simulink model "SecRwRtStCaller"  (R2018b)
settings: Solver=FixedStepDiscrete  StartTime=0.0  StopTime=10.0  RelTol=1e-3
undefined symbols (not defined in the file or in its folder): SecRwRtStArmScrnCtrl_1_Cal, SecRwRtStArmScrnHolderChk_1_Cal, SecRwRtStArmScrnIsPosChk_1_Cal, SecRwRtStArmScrnTrgtPosSelc_1_Cal, SecRwRtStBkReclnCtrl_1_Cal, SecRwRtStBkReclnHolderChk_1_Cal, SecRwRtStBkReclnIsPosChk_1_Cal, SecRwRtStBkReclnTrgtPosSelc_1_Cal, SecRwRtStChldLckChk_Cal, SecRwRtStFtrstCtrl_1_Cal, SecRwRtStFtrstHolderChk_1_Cal, SecRwRtStFtrstIsPosChk_1_Cal, SecRwRtStFtrstTrgtPosSelc_1_Cal, SecRwRtStFwdBkwdCtrl_1_Cal, SecRwRtStFwdBkwdHolderChk_1_Cal, SecRwRtStFwdBkwdIsPosChk_1_Cal, SecRwRtStFwdBkwdSpdCtrl_1_Cal, SecRwRtStFwdBkwdTrgtPosSelc_1_Cal, SecRwRtStHdrstFwdBkwdCtrl_1_Cal, SecRwRtStHdrstFwdBkwdHolderChk_1_Cal, SecRwRtStHdrstFwdBkwdIsPosChk_1_Cal, SecRwRtStHdrstFwdBkwdTrgtPosSelc_1_Cal, SecRwRtStHdrstUpwdDnwdCtrl_1_Cal, SecRwRtStHdrstUpwdDnwdHolderChk_1_Cal, SecRwRtStHdrstUpwdDnwdIsPosChk_1_Cal, SecRwRtStHdrstUpwdDnwdTrgtPosSelc_1_Cal, SecRwRtStHeightChk_Cal, SecRwRtStLgrstInwdOtwdCtrl_1_Cal, SecRwRtStLgrstInwdOtwdHolderChk_1_Cal, SecRwRtStLgrstInwdOtwdIsPosChk_1_Cal, SecRwRtStLgrstInwdOtwdTrgtPosSelc_1_Cal, SecRwRtStLgrstUpwdDnwdCtrl_1_Cal, SecRwRtStLgrstUpwdDnwdHolderChk_1_Cal, SecRwRtStLgrstUpwdDnwdIsPosChk_1_Cal, SecRwRtStLgrstUpwdDnwdTrgtPosSelc_1_Cal, SecRwRtStLtwdRtwdCtrl_1_Cal, SecRwRtStLtwdRtwdHolderChk_1_Cal, SecRwRtStLtwdRtwdIsPosChk_1_Cal, SecRwRtStLtwdRtwdTrgtPosSelc_1_Cal, SecRwRtStOccupyChk_Cal, SecRwRtStRclCmdSrvCal_1_Cal, SecRwRtStZeroCtrl_1_Cal, SecRwRtStZeroHolderChk_1_Cal, SecRwRtStZeroIsPosChk_1_Cal, SecRwRtStZeroTrgtPosSelc_1_Cal
settings Model: Creator=sn2xws  LastModifiedBy=sn2xws
settings Model: ModifiedHistory=|
  | 2024.5.6
  | 557 新增零重力电机
settings DataIOCC: SaveFormat=StructureWithTime
settings OptimizationCC: DefaultParameterBehavior=Inlined  EnhancedBackFolding=on  PassReuseOutputArgsAs=Individual arguments  ZeroExternalMemoryAtStartup=off  ZeroInternalMemoryAtStartup=off  OptimizeBlockOrder=speed  DifferentSizesBufferReuse=on  OptimizationCustomize=off
settings DebuggingCC: ParameterTunabilityLossMsg=error
settings SFSimCC: MATLABDynamicMemAlloc=off
settings RTWCC: SystemTargetFile=autosar.tlc  GenCodeOnly=on  TemplateMakefile=ert_default_tmf  Description=AUTOSAR  GenerateReport=on  IncludeHyperlinkInReport=on  LaunchReport=on  GenerateTraceInfo=on  GenerateTraceReport=on  GenerateTraceReportSl=on  GenerateTraceReportSf=on  GenerateTraceReportEml=on
settings CodeAppCC: ForceParamTrailComments=on  IgnoreCustomStorageClasses=off  OperatorAnnotations=on  SimulinkDataObjDesc=on  SFDataObjDesc=on  InsertBlockDesc=on
settings STFCustomTargetCC: TargetLangStandard=C99 (ISO)  MultiwordLength=256  ParMdlRefBuildCompliant=on  CompOptLevelCompliant=on  IncludeMdlTerminateFcn=off  CombineOutputUpdateFcns=on  SuppressErrorStatus=on  ERTCustomFileBanners=on  SupportNonFinite=off  SupportComplex=off  SupportContinuousTime=off  SupportNonInlinedSFcns=off  RemoveResetFunc=on  MATLABClassNameForMDSCustomization=Simulink.SoftwareTarget.ERTCustomization  AutosarCompliant=on  UseToolchainInfoCompliant=on  LookupTableObjectStructAxisOrder=2,1,3,4,...  LUTObjectStructOrderEvenSpacing=Size,Table,Breakpoints  SystemTargetFile=autosar.tlc
settings ERTTargetCC: TargetLangStandard=C99 (ISO)  ConcurrentExecutionCompliant=off  IncludeMdlTerminateFcn=off  SuppressErrorStatus=on  SupportNonFinite=off  SupportComplex=off  ModelStepFunctionPrototypeControlCompliant=off  CPPClassGenCompliant=off  AutosarCompliant=on  LookupTableObjectStructAxisOrder=2,1,3,4,...  LUTObjectStructOrderEvenSpacing=Size,Table,Breakpoints  InlinedParameterPlacement=NonHierarchical  ERTCustomFileTemplate=example_file_process.tlc  ERTFilePackagingFormat=Compact

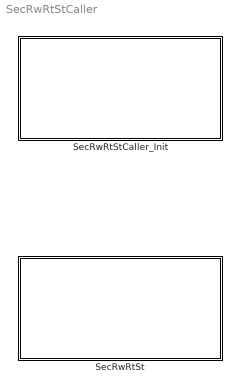
== system SecRwRtStCaller ==
  SecRwRtSt : Subsystem
  SecRwRtStCaller_Init : Subsystem

== system SecRwRtStCaller/SecRwRtSt ==
  SecRwRtSt_Cal_sys : Subsystem

== system SecRwRtStCaller/SecRwRtStCaller_Init ==
  Event Listener : EventListener  EventName=reset

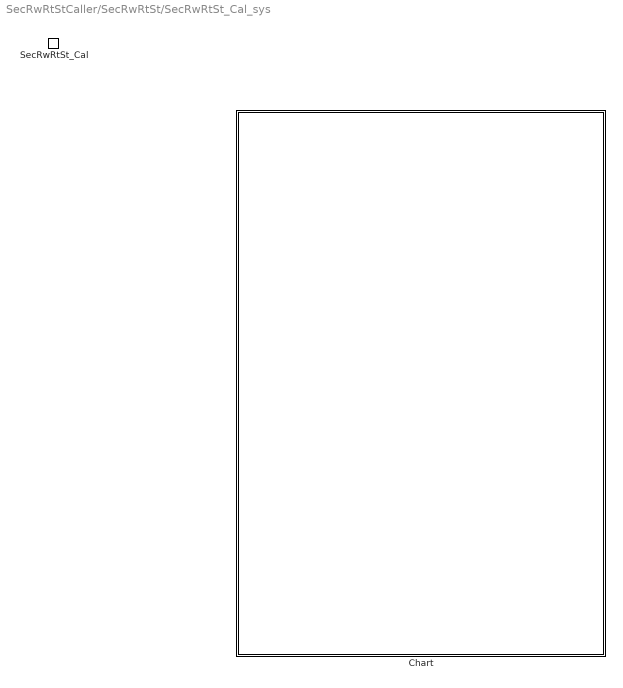
== system SecRwRtStCaller/SecRwRtSt/SecRwRtSt_Cal_sys ==
  SecRwRtSt_Cal : TriggerPort  TriggerType=function-call  IsSimulinkFunction=on  FunctionName=SecRwRtSt_Cal  VariantControl=(inherit)
  Chart : Stateflow chart  TreatAsAtomicUnit=on

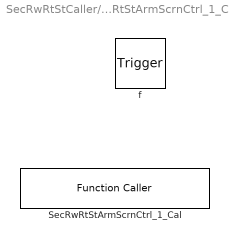
== system SecRwRtStCaller/SecRwRtSt/SecRwRtSt_Cal_sys/Chart/SecRwRtStArmScrnCtrl_1_Cal ==
  f : TriggerPort  TriggerType=function-call  VariantControl=(inherit)
      settings: CopyFcn=Stateflow.SLINSF.SimulinkMan.removeBlockPreDeleteFcn  PreDeleteFcn=Stateflow.SLINSF.SimulinkMan.unsafePredeleteFcn
  SecRwRtStArmScrnCtrl_1_Cal : FunctionCaller  FunctionPrototype=SecRwRtStArmScrnCtrl_1_Cal()

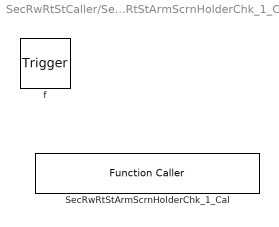
== system SecRwRtStCaller/SecRwRtSt/SecRwRtSt_Cal_sys/Chart/SecRwRtStArmScrnHolderChk_1_Cal ==
  f : TriggerPort  TriggerType=function-call  VariantControl=(inherit)
      settings: CopyFcn=Stateflow.SLINSF.SimulinkMan.removeBlockPreDeleteFcn  PreDeleteFcn=Stateflow.SLINSF.SimulinkMan.unsafePredeleteFcn
  SecRwRtStArmScrnHolderChk_1_Cal : FunctionCaller  FunctionPrototype=SecRwRtStArmScrnHolderChk_1_Cal()

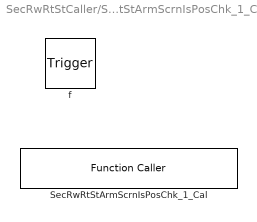
== system SecRwRtStCaller/SecRwRtSt/SecRwRtSt_Cal_sys/Chart/SecRwRtStArmScrnIsPosChk_1_Cal ==
  f : TriggerPort  TriggerType=function-call  VariantControl=(inherit)
      settings: CopyFcn=Stateflow.SLINSF.SimulinkMan.removeBlockPreDeleteFcn  PreDeleteFcn=Stateflow.SLINSF.SimulinkMan.unsafePredeleteFcn
  SecRwRtStArmScrnIsPosChk_1_Cal : FunctionCaller  FunctionPrototype=SecRwRtStArmScrnIsPosChk_1_Cal()

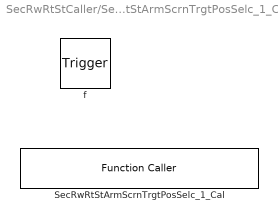
== system SecRwRtStCaller/SecRwRtSt/SecRwRtSt_Cal_sys/Chart/SecRwRtStArmScrnTrgtPosSelc_1_Cal ==
  f : TriggerPort  TriggerType=function-call  VariantControl=(inherit)
      settings: CopyFcn=Stateflow.SLINSF.SimulinkMan.removeBlockPreDeleteFcn  PreDeleteFcn=Stateflow.SLINSF.SimulinkMan.unsafePredeleteFcn
  SecRwRtStArmScrnTrgtPosSelc_1_Cal : FunctionCaller  FunctionPrototype=SecRwRtStArmScrnTrgtPosSelc_1_Cal()

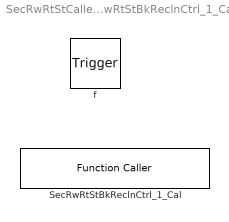
== system SecRwRtStCaller/SecRwRtSt/SecRwRtSt_Cal_sys/Chart/SecRwRtStBkReclnCtrl_1_Cal ==
  f : TriggerPort  TriggerType=function-call  VariantControl=(inherit)
      settings: CopyFcn=Stateflow.SLINSF.SimulinkMan.removeBlockPreDeleteFcn  PreDeleteFcn=Stateflow.SLINSF.SimulinkMan.unsafePredeleteFcn
  SecRwRtStBkReclnCtrl_1_Cal : FunctionCaller  FunctionPrototype=SecRwRtStBkReclnCtrl_1_Cal()

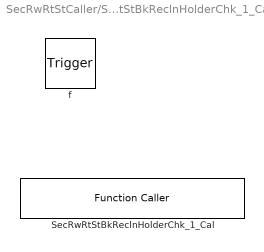
== system SecRwRtStCaller/SecRwRtSt/SecRwRtSt_Cal_sys/Chart/SecRwRtStBkReclnHolderChk_1_Cal ==
  f : TriggerPort  TriggerType=function-call  VariantControl=(inherit)
      settings: CopyFcn=Stateflow.SLINSF.SimulinkMan.removeBlockPreDeleteFcn  PreDeleteFcn=Stateflow.SLINSF.SimulinkMan.unsafePredeleteFcn
  SecRwRtStBkReclnHolderChk_1_Cal : FunctionCaller  FunctionPrototype=SecRwRtStBkReclnHolderChk_1_Cal()

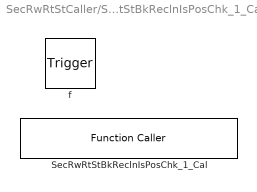
== system SecRwRtStCaller/SecRwRtSt/SecRwRtSt_Cal_sys/Chart/SecRwRtStBkReclnIsPosChk_1_Cal ==
  f : TriggerPort  TriggerType=function-call  VariantControl=(inherit)
      settings: CopyFcn=Stateflow.SLINSF.SimulinkMan.removeBlockPreDeleteFcn  PreDeleteFcn=Stateflow.SLINSF.SimulinkMan.unsafePredeleteFcn
  SecRwRtStBkReclnIsPosChk_1_Cal : FunctionCaller  FunctionPrototype=SecRwRtStBkReclnIsPosChk_1_Cal()

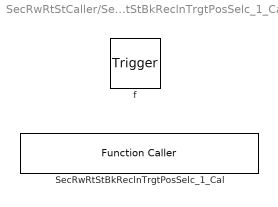
== system SecRwRtStCaller/SecRwRtSt/SecRwRtSt_Cal_sys/Chart/SecRwRtStBkReclnTrgtPosSelc_1_Cal ==
  f : TriggerPort  TriggerType=function-call  VariantControl=(inherit)
      settings: CopyFcn=Stateflow.SLINSF.SimulinkMan.removeBlockPreDeleteFcn  PreDeleteFcn=Stateflow.SLINSF.SimulinkMan.unsafePredeleteFcn
  SecRwRtStBkReclnTrgtPosSelc_1_Cal : FunctionCaller  FunctionPrototype=SecRwRtStBkReclnTrgtPosSelc_1_Cal()

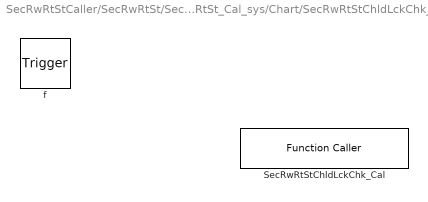
== system SecRwRtStCaller/SecRwRtSt/SecRwRtSt_Cal_sys/Chart/SecRwRtStChldLckChk_Cal ==
  f : TriggerPort  TriggerType=function-call  VariantControl=(inherit)
      settings: CopyFcn=Stateflow.SLINSF.SimulinkMan.removeBlockPreDeleteFcn  PreDeleteFcn=Stateflow.SLINSF.SimulinkMan.unsafePredeleteFcn
  SecRwRtStChldLckChk_Cal : FunctionCaller  FunctionPrototype=SecRwRtStChldLckChk_Cal()

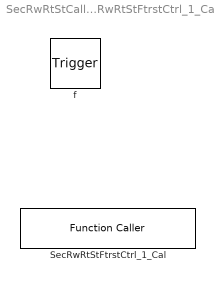
== system SecRwRtStCaller/SecRwRtSt/SecRwRtSt_Cal_sys/Chart/SecRwRtStFtrstCtrl_1_Cal ==
  f : TriggerPort  TriggerType=function-call  VariantControl=(inherit)
      settings: CopyFcn=Stateflow.SLINSF.SimulinkMan.removeBlockPreDeleteFcn  PreDeleteFcn=Stateflow.SLINSF.SimulinkMan.unsafePredeleteFcn
  SecRwRtStFtrstCtrl_1_Cal : FunctionCaller  FunctionPrototype=SecRwRtStFtrstCtrl_1_Cal()

== system SecRwRtStCaller/SecRwRtSt/SecRwRtSt_Cal_sys/Chart/SecRwRtStFtrstHolderChk_1_Cal ==
  f : TriggerPort  TriggerType=function-call  VariantControl=(inherit)
      settings: CopyFcn=Stateflow.SLINSF.SimulinkMan.removeBlockPreDeleteFcn  PreDeleteFcn=Stateflow.SLINSF.SimulinkMan.unsafePredeleteFcn
  SecRwRtStFtrstHolderChk_1_Cal : FunctionCaller  FunctionPrototype=SecRwRtStFtrstHolderChk_1_Cal()

== system SecRwRtStCaller/SecRwRtSt/SecRwRtSt_Cal_sys/Chart/SecRwRtStFtrstIsPosChk_1_Cal ==
  f : TriggerPort  TriggerType=function-call  VariantControl=(inherit)
      settings: CopyFcn=Stateflow.SLINSF.SimulinkMan.removeBlockPreDeleteFcn  PreDeleteFcn=Stateflow.SLINSF.SimulinkMan.unsafePredeleteFcn
  SecRwRtStFtrstIsPosChk_1_Cal : FunctionCaller  FunctionPrototype=SecRwRtStFtrstIsPosChk_1_Cal()

== system SecRwRtStCaller/SecRwRtSt/SecRwRtSt_Cal_sys/Chart/SecRwRtStFtrstTrgtPosSelc_1_Cal ==
  f : TriggerPort  TriggerType=function-call  VariantControl=(inherit)
      settings: CopyFcn=Stateflow.SLINSF.SimulinkMan.removeBlockPreDeleteFcn  PreDeleteFcn=Stateflow.SLINSF.SimulinkMan.unsafePredeleteFcn
  SecRwRtStFtrstTrgtPosSelc_1_Cal : FunctionCaller  FunctionPrototype=SecRwRtStFtrstTrgtPosSelc_1_Cal()

== system SecRwRtStCaller/SecRwRtSt/SecRwRtSt_Cal_sys/Chart/SecRwRtStFwdBkwdCtrl_1_Cal ==
  f : TriggerPort  TriggerType=function-call  VariantControl=(inherit)
      settings: CopyFcn=Stateflow.SLINSF.SimulinkMan.removeBlockPreDeleteFcn  PreDeleteFcn=Stateflow.SLINSF.SimulinkMan.unsafePredeleteFcn
  SecRwRtStFwdBkwdCtrl_1_Cal : FunctionCaller  FunctionPrototype=SecRwRtStFwdBkwdCtrl_1_Cal()

== system SecRwRtStCaller/SecRwRtSt/SecRwRtSt_Cal_sys/Chart/SecRwRtStFwdBkwdHolderChk_1_Cal ==
  f : TriggerPort  TriggerType=function-call  VariantControl=(inherit)
      settings: CopyFcn=Stateflow.SLINSF.SimulinkMan.removeBlockPreDeleteFcn  PreDeleteFcn=Stateflow.SLINSF.SimulinkMan.unsafePredeleteFcn
  SecRwRtStFwdBkwdHolderChk_1_Cal : FunctionCaller  FunctionPrototype=SecRwRtStFwdBkwdHolderChk_1_Cal()

== system SecRwRtStCaller/SecRwRtSt/SecRwRtSt_Cal_sys/Chart/SecRwRtStFwdBkwdIsPosChk_1_Cal ==
  f : TriggerPort  TriggerType=function-call  VariantControl=(inherit)
      settings: CopyFcn=Stateflow.SLINSF.SimulinkMan.removeBlockPreDeleteFcn  PreDeleteFcn=Stateflow.SLINSF.SimulinkMan.unsafePredeleteFcn
  SecRwRtStFwdBkwdIsPosChk_1_Cal : FunctionCaller  FunctionPrototype=SecRwRtStFwdBkwdIsPosChk_1_Cal()

== system SecRwRtStCaller/SecRwRtSt/SecRwRtSt_Cal_sys/Chart/SecRwRtStFwdBkwdSpdCtrl_1_Cal ==
  f : TriggerPort  TriggerType=function-call  VariantControl=(inherit)
      settings: CopyFcn=Stateflow.SLINSF.SimulinkMan.removeBlockPreDeleteFcn  PreDeleteFcn=Stateflow.SLINSF.SimulinkMan.unsafePredeleteFcn
  SecRwRtStFwdBkwdSpdCtrl_1_Cal : FunctionCaller  FunctionPrototype=SecRwRtStFwdBkwdSpdCtrl_1_Cal()

== system SecRwRtStCaller/SecRwRtSt/SecRwRtSt_Cal_sys/Chart/SecRwRtStFwdBkwdTrgtPosSelc_1_Cal ==
  f : TriggerPort  TriggerType=function-call  VariantControl=(inherit)
      settings: CopyFcn=Stateflow.SLINSF.SimulinkMan.removeBlockPreDeleteFcn  PreDeleteFcn=Stateflow.SLINSF.SimulinkMan.unsafePredeleteFcn
  SecRwRtStFwdBkwdTrgtPosSelc_1_Cal : FunctionCaller  FunctionPrototype=SecRwRtStFwdBkwdTrgtPosSelc_1_Cal()

== system SecRwRtStCaller/SecRwRtSt/SecRwRtSt_Cal_sys/Chart/SecRwRtStHdrstFwdBkwdCtrl_1_Cal ==
  f : TriggerPort  TriggerType=function-call  VariantControl=(inherit)
      settings: CopyFcn=Stateflow.SLINSF.SimulinkMan.removeBlockPreDeleteFcn  PreDeleteFcn=Stateflow.SLINSF.SimulinkMan.unsafePredeleteFcn
  SecRwRtStHdrstFwdBkwdCtrl_1_Cal : FunctionCaller  FunctionPrototype=SecRwRtStHdrstFwdBkwdCtrl_1_Cal()

== system SecRwRtStCaller/SecRwRtSt/SecRwRtSt_Cal_sys/Chart/SecRwRtStHdrstFwdBkwdHolderChk_1_Cal ==
  f : TriggerPort  TriggerType=function-call  VariantControl=(inherit)
      settings: CopyFcn=Stateflow.SLINSF.SimulinkMan.removeBlockPreDeleteFcn  PreDeleteFcn=Stateflow.SLINSF.SimulinkMan.unsafePredeleteFcn
  SecRwRtStHdrstFwdBkwdHolderChk_1_Cal : FunctionCaller  FunctionPrototype=SecRwRtStHdrstFwdBkwdHolderChk_1_Cal()

== system SecRwRtStCaller/SecRwRtSt/SecRwRtSt_Cal_sys/Chart/SecRwRtStHdrstFwdBkwdIsPosChk_1_Cal ==
  f : TriggerPort  TriggerType=function-call  VariantControl=(inherit)
      settings: CopyFcn=Stateflow.SLINSF.SimulinkMan.removeBlockPreDeleteFcn  PreDeleteFcn=Stateflow.SLINSF.SimulinkMan.unsafePredeleteFcn
  SecRwRtStHdrstFwdBkwdIsPosChk_1_Cal : FunctionCaller  FunctionPrototype=SecRwRtStHdrstFwdBkwdIsPosChk_1_Cal()

== system SecRwRtStCaller/SecRwRtSt/SecRwRtSt_Cal_sys/Chart/SecRwRtStHdrstFwdBkwdTrgtPosSelc_1_Cal ==
  f : TriggerPort  TriggerType=function-call  VariantControl=(inherit)
      settings: CopyFcn=Stateflow.SLINSF.SimulinkMan.removeBlockPreDeleteFcn  PreDeleteFcn=Stateflow.SLINSF.SimulinkMan.unsafePredeleteFcn
  SecRwRtStHdrstFwdBkwdTrgtPosSelc_1_Cal : FunctionCaller  FunctionPrototype=SecRwRtStHdrstFwdBkwdTrgtPosSelc_1_Cal()

== system SecRwRtStCaller/SecRwRtSt/SecRwRtSt_Cal_sys/Chart/SecRwRtStHdrstUpwdDnwdCtrl_1_Cal ==
  f : TriggerPort  TriggerType=function-call  VariantControl=(inherit)
      settings: CopyFcn=Stateflow.SLINSF.SimulinkMan.removeBlockPreDeleteFcn  PreDeleteFcn=Stateflow.SLINSF.SimulinkMan.unsafePredeleteFcn
  SecRwRtStHdrstUpwdDnwdCtrl_1_Cal : FunctionCaller  FunctionPrototype=SecRwRtStHdrstUpwdDnwdCtrl_1_Cal()

== system SecRwRtStCaller/SecRwRtSt/SecRwRtSt_Cal_sys/Chart/SecRwRtStHdrstUpwdDnwdHolderChk_1_Cal ==
  f : TriggerPort  TriggerType=function-call  VariantControl=(inherit)
      settings: CopyFcn=Stateflow.SLINSF.SimulinkMan.removeBlockPreDeleteFcn  PreDeleteFcn=Stateflow.SLINSF.SimulinkMan.unsafePredeleteFcn
  SecRwRtStHdrstUpwdDnwdHolderChk_1_Cal : FunctionCaller  FunctionPrototype=SecRwRtStHdrstUpwdDnwdHolderChk_1_Cal()

== system SecRwRtStCaller/SecRwRtSt/SecRwRtSt_Cal_sys/Chart/SecRwRtStHdrstUpwdDnwdIsPosChk_1_Cal ==
  f : TriggerPort  TriggerType=function-call  VariantControl=(inherit)
      settings: CopyFcn=Stateflow.SLINSF.SimulinkMan.removeBlockPreDeleteFcn  PreDeleteFcn=Stateflow.SLINSF.SimulinkMan.unsafePredeleteFcn
  SecRwRtStHdrstUpwdDnwdIsPosChk_1_Cal : FunctionCaller  FunctionPrototype=SecRwRtStHdrstUpwdDnwdIsPosChk_1_Cal()

== system SecRwRtStCaller/SecRwRtSt/SecRwRtSt_Cal_sys/Chart/SecRwRtStHdrstUpwdDnwdTrgtPosSelc_1_Cal ==
  f : TriggerPort  TriggerType=function-call  VariantControl=(inherit)
      settings: CopyFcn=Stateflow.SLINSF.SimulinkMan.removeBlockPreDeleteFcn  PreDeleteFcn=Stateflow.SLINSF.SimulinkMan.unsafePredeleteFcn
  SecRwRtStHdrstUpwdDnwdTrgtPosSelc_1_Cal : FunctionCaller  FunctionPrototype=SecRwRtStHdrstUpwdDnwdTrgtPosSelc_1_Cal()

== system SecRwRtStCaller/SecRwRtSt/SecRwRtSt_Cal_sys/Chart/SecRwRtStHeightChk_Cal ==
  f : TriggerPort  TriggerType=function-call  VariantControl=(inherit)
      settings: CopyFcn=Stateflow.SLINSF.SimulinkMan.removeBlockPreDeleteFcn  PreDeleteFcn=Stateflow.SLINSF.SimulinkMan.unsafePredeleteFcn
  SecRwRtStHeightChk_Cal : FunctionCaller  FunctionPrototype=SecRwRtStHeightChk_Cal()

== system SecRwRtStCaller/SecRwRtSt/SecRwRtSt_Cal_sys/Chart/SecRwRtStLgrstInwdOtwdCtrl_1_Cal ==
  f : TriggerPort  TriggerType=function-call  VariantControl=(inherit)
      settings: CopyFcn=Stateflow.SLINSF.SimulinkMan.removeBlockPreDeleteFcn  PreDeleteFcn=Stateflow.SLINSF.SimulinkMan.unsafePredeleteFcn
  SecRwRtStLgrstInwdOtwdCtrl_1_Cal : FunctionCaller  FunctionPrototype=SecRwRtStLgrstInwdOtwdCtrl_1_Cal()

== system SecRwRtStCaller/SecRwRtSt/SecRwRtSt_Cal_sys/Chart/SecRwRtStLgrstInwdOtwdHolderChk_1_Cal ==
  f : TriggerPort  TriggerType=function-call  VariantControl=(inherit)
      settings: CopyFcn=Stateflow.SLINSF.SimulinkMan.removeBlockPreDeleteFcn  PreDeleteFcn=Stateflow.SLINSF.SimulinkMan.unsafePredeleteFcn
  SecRwRtStLgrstInwdOtwdHolderChk_1_Cal : FunctionCaller  FunctionPrototype=SecRwRtStLgrstInwdOtwdHolderChk_1_Cal()

== system SecRwRtStCaller/SecRwRtSt/SecRwRtSt_Cal_sys/Chart/SecRwRtStLgrstInwdOtwdIsPosChk_1_Cal ==
  f : TriggerPort  TriggerType=function-call  VariantControl=(inherit)
      settings: CopyFcn=Stateflow.SLINSF.SimulinkMan.removeBlockPreDeleteFcn  PreDeleteFcn=Stateflow.SLINSF.SimulinkMan.unsafePredeleteFcn
  SecRwRtStLgrstInwdOtwdIsPosChk_1_Cal : FunctionCaller  FunctionPrototype=SecRwRtStLgrstInwdOtwdIsPosChk_1_Cal()

== system SecRwRtStCaller/SecRwRtSt/SecRwRtSt_Cal_sys/Chart/SecRwRtStLgrstInwdOtwdTrgtPosSelc_1_Cal ==
  f : TriggerPort  TriggerType=function-call  VariantControl=(inherit)
      settings: CopyFcn=Stateflow.SLINSF.SimulinkMan.removeBlockPreDeleteFcn  PreDeleteFcn=Stateflow.SLINSF.SimulinkMan.unsafePredeleteFcn
  SecRwRtStLgrstInwdOtwdTrgtPosSelc_1_Cal : FunctionCaller  FunctionPrototype=SecRwRtStLgrstInwdOtwdTrgtPosSelc_1_Cal()

== system SecRwRtStCaller/SecRwRtSt/SecRwRtSt_Cal_sys/Chart/SecRwRtStLgrstUpwdDnwdCtrl_1_Cal ==
  f : TriggerPort  TriggerType=function-call  VariantControl=(inherit)
      settings: CopyFcn=Stateflow.SLINSF.SimulinkMan.removeBlockPreDeleteFcn  PreDeleteFcn=Stateflow.SLINSF.SimulinkMan.unsafePredeleteFcn
  SecRwRtStLgrstUpwdDnwdCtrl_1_Cal : FunctionCaller  FunctionPrototype=SecRwRtStLgrstUpwdDnwdCtrl_1_Cal()

== system SecRwRtStCaller/SecRwRtSt/SecRwRtSt_Cal_sys/Chart/SecRwRtStLgrstUpwdDnwdHolderChk_1_Cal ==
  f : TriggerPort  TriggerType=function-call  VariantControl=(inherit)
      settings: CopyFcn=Stateflow.SLINSF.SimulinkMan.removeBlockPreDeleteFcn  PreDeleteFcn=Stateflow.SLINSF.SimulinkMan.unsafePredeleteFcn
  SecRwRtStLgrstUpwdDnwdHolderChk_1_Cal : FunctionCaller  FunctionPrototype=SecRwRtStLgrstUpwdDnwdHolderChk_1_Cal()

== system SecRwRtStCaller/SecRwRtSt/SecRwRtSt_Cal_sys/Chart/SecRwRtStLgrstUpwdDnwdIsPosChk_1_Cal ==
  f : TriggerPort  TriggerType=function-call  VariantControl=(inherit)
      settings: CopyFcn=Stateflow.SLINSF.SimulinkMan.removeBlockPreDeleteFcn  PreDeleteFcn=Stateflow.SLINSF.SimulinkMan.unsafePredeleteFcn
  SecRwRtStLgrstUpwdDnwdIsPosChk_1_Cal : FunctionCaller  FunctionPrototype=SecRwRtStLgrstUpwdDnwdIsPosChk_1_Cal()

== system SecRwRtStCaller/SecRwRtSt/SecRwRtSt_Cal_sys/Chart/SecRwRtStLgrstUpwdDnwdTrgtPosSelc_1_Cal ==
  f : TriggerPort  TriggerType=function-call  VariantControl=(inherit)
      settings: CopyFcn=Stateflow.SLINSF.SimulinkMan.removeBlockPreDeleteFcn  PreDeleteFcn=Stateflow.SLINSF.SimulinkMan.unsafePredeleteFcn
  SecRwRtStLgrstUpwdDnwdTrgtPosSelc_1_Cal : FunctionCaller  FunctionPrototype=SecRwRtStLgrstUpwdDnwdTrgtPosSelc_1_Cal()

== system SecRwRtStCaller/SecRwRtSt/SecRwRtSt_Cal_sys/Chart/SecRwRtStLtwdRtwdCtrl_1_Cal ==
  f : TriggerPort  TriggerType=function-call  VariantControl=(inherit)
      settings: CopyFcn=Stateflow.SLINSF.SimulinkMan.removeBlockPreDeleteFcn  PreDeleteFcn=Stateflow.SLINSF.SimulinkMan.unsafePredeleteFcn
  SecRwRtStLtwdRtwdCtrl_1_Cal : FunctionCaller  FunctionPrototype=SecRwRtStLtwdRtwdCtrl_1_Cal()

== system SecRwRtStCaller/SecRwRtSt/SecRwRtSt_Cal_sys/Chart/SecRwRtStLtwdRtwdHolderChk_1_Cal ==
  f : TriggerPort  TriggerType=function-call  VariantControl=(inherit)
      settings: CopyFcn=Stateflow.SLINSF.SimulinkMan.removeBlockPreDeleteFcn  PreDeleteFcn=Stateflow.SLINSF.SimulinkMan.unsafePredeleteFcn
  SecRwRtStLtwdRtwdHolderChk_1_Cal : FunctionCaller  FunctionPrototype=SecRwRtStLtwdRtwdHolderChk_1_Cal()

== system SecRwRtStCaller/SecRwRtSt/SecRwRtSt_Cal_sys/Chart/SecRwRtStLtwdRtwdIsPosChk_1_Cal ==
  f : TriggerPort  TriggerType=function-call  VariantControl=(inherit)
      settings: CopyFcn=Stateflow.SLINSF.SimulinkMan.removeBlockPreDeleteFcn  PreDeleteFcn=Stateflow.SLINSF.SimulinkMan.unsafePredeleteFcn
  SecRwRtStLtwdRtwdIsPosChk_1_Cal : FunctionCaller  FunctionPrototype=SecRwRtStLtwdRtwdIsPosChk_1_Cal()

== system SecRwRtStCaller/SecRwRtSt/SecRwRtSt_Cal_sys/Chart/SecRwRtStLtwdRtwdTrgtPosSelc_1_Cal ==
  f : TriggerPort  TriggerType=function-call  VariantControl=(inherit)
      settings: CopyFcn=Stateflow.SLINSF.SimulinkMan.removeBlockPreDeleteFcn  PreDeleteFcn=Stateflow.SLINSF.SimulinkMan.unsafePredeleteFcn
  SecRwRtStLtwdRtwdTrgtPosSelc_1_Cal : FunctionCaller  FunctionPrototype=SecRwRtStLtwdRtwdTrgtPosSelc_1_Cal()

== system SecRwRtStCaller/SecRwRtSt/SecRwRtSt_Cal_sys/Chart/SecRwRtStOccupyChk_Cal ==
  f : TriggerPort  TriggerType=function-call  VariantControl=(inherit)
      settings: CopyFcn=Stateflow.SLINSF.SimulinkMan.removeBlockPreDeleteFcn  PreDeleteFcn=Stateflow.SLINSF.SimulinkMan.unsafePredeleteFcn
  SecRwRtStOccupyChk_Cal : FunctionCaller  FunctionPrototype=SecRwRtStOccupyChk_Cal()

== system SecRwRtStCaller/SecRwRtSt/SecRwRtSt_Cal_sys/Chart/SecRwRtStRclCmdSrvCal_1_Cal ==
  f : TriggerPort  TriggerType=function-call  VariantControl=(inherit)
      settings: CopyFcn=Stateflow.SLINSF.SimulinkMan.removeBlockPreDeleteFcn  PreDeleteFcn=Stateflow.SLINSF.SimulinkMan.unsafePredeleteFcn
  SecRwRtStRclCmdSrvCal_1_Cal : FunctionCaller  FunctionPrototype=SecRwRtStRclCmdSrvCal_1_Cal()

== system SecRwRtStCaller/SecRwRtSt/SecRwRtSt_Cal_sys/Chart/SecRwRtStZeroCtrl_1_Cal ==
  f : TriggerPort  TriggerType=function-call  VariantControl=(inherit)
      settings: CopyFcn=Stateflow.SLINSF.SimulinkMan.removeBlockPreDeleteFcn  PreDeleteFcn=Stateflow.SLINSF.SimulinkMan.unsafePredeleteFcn
  SecRwRtStZeroCtrl_1_Cal : FunctionCaller  FunctionPrototype=SecRwRtStZeroCtrl_1_Cal()

== system SecRwRtStCaller/SecRwRtSt/SecRwRtSt_Cal_sys/Chart/SecRwRtStZeroHolderChk_1_Cal ==
  f : TriggerPort  TriggerType=function-call  VariantControl=(inherit)
      settings: CopyFcn=Stateflow.SLINSF.SimulinkMan.removeBlockPreDeleteFcn  PreDeleteFcn=Stateflow.SLINSF.SimulinkMan.unsafePredeleteFcn
  SecRwRtStZeroHolderChk_1_Cal : FunctionCaller  FunctionPrototype=SecRwRtStZeroHolderChk_1_Cal()

== system SecRwRtStCaller/SecRwRtSt/SecRwRtSt_Cal_sys/Chart/SecRwRtStZeroIsPosChk_1_Cal ==
  f : TriggerPort  TriggerType=function-call  VariantControl=(inherit)
      settings: CopyFcn=Stateflow.SLINSF.SimulinkMan.removeBlockPreDeleteFcn  PreDeleteFcn=Stateflow.SLINSF.SimulinkMan.unsafePredeleteFcn
  SecRwRtStZeroIsPosChk_1_Cal : FunctionCaller  FunctionPrototype=SecRwRtStZeroIsPosChk_1_Cal()

== system SecRwRtStCaller/SecRwRtSt/SecRwRtSt_Cal_sys/Chart/SecRwRtStZeroTrgtPosSelc_1_Cal ==
  f : TriggerPort  TriggerType=function-call  VariantControl=(inherit)
      settings: CopyFcn=Stateflow.SLINSF.SimulinkMan.removeBlockPreDeleteFcn  PreDeleteFcn=Stateflow.SLINSF.SimulinkMan.unsafePredeleteFcn
  SecRwRtStZeroTrgtPosSelc_1_Cal : FunctionCaller  FunctionPrototype=SecRwRtStZeroTrgtPosSelc_1_Cal()

== stateflow chart SecRwRtStCaller/SecRwRtSt/SecRwRtSt_Cal_sys/Chart ==
  state SecRwRtStArmScrnCtrl_1_Cal [function]
  state SecRwRtStBkReclnCtrl_1_Cal [function]
  state SecRwRtStFtrstCtrl_1_Cal [function]
  state SecRwRtStChldLckChk_Cal [function]
  state SecRwRtStArmScrnHolderChk_1_Cal [function]
  state SecRwRtStBkReclnHolderChk_1_Cal [function]
  state SecRwRtStFtrstHolderChk_1_Cal [function]
  state SecRwRtStFwdBkwdSpdCtrl_1_Cal [function]
  state SecRwRtStArmScrnIsPosChk_1_Cal [function]
  state SecRwRtStBkReclnIsPosChk_1_Cal [function]
  state SecRwRtStFtrstIsPosChk_1_Cal [function]
  state SecRwRtStHeightChk_Cal [function]
  state SecRwRtStArmScrnTrgtPosSelc_1_Cal [function]
  state SecRwRtStBkReclnTrgtPosSelc_1_Cal [function]
  state SecRwRtStFtrstTrgtPosSelc_1_Cal [function]
  state SecRwRtStOccupyChk_Cal [function]
  state SecRwRtStRclCmdSrvCal_1_Cal [function]
  state SecRwRtStFwdBkwdCtrl_1_Cal [function]
  state SecRwRtStHdrstFwdBkwdCtrl_1_Cal [function]
  state SecRwRtStHdrstUpwdDnwdCtrl_1_Cal [function]
  state SecRwRtStFwdBkwdHolderChk_1_Cal [function]
  state SecRwRtStHdrstFwdBkwdHolderChk_1_Cal [function]
  state SecRwRtStHdrstUpwdDnwdHolderChk_1_Cal [function]
  state SecRwRtStFwdBkwdIsPosChk_1_Cal [function]
  state SecRwRtStHdrstFwdBkwdIsPosChk_1_Cal [function]
  state SecRwRtStHdrstUpwdDnwdIsPosChk_1_Cal [function]
  state SecRwRtStFwdBkwdTrgtPosSelc_1_Cal [function]
  state SecRwRtStHdrstFwdBkwdTrgtPosSelc_1_Cal [function]
  state SecRwRtStHdrstUpwdDnwdTrgtPosSelc_1_Cal [function]
  state SecRwRtStLgrstInwdOtwdCtrl_1_Cal [function]
  state SecRwRtStLgrstUpwdDnwdCtrl_1_Cal [function]
  state SecRwRtStLtwdRtwdCtrl_1_Cal [function]
  state SecRwRtStLgrstInwdOtwdHolderChk_1_Cal [function]
  state SecRwRtStLgrstUpwdDnwdHolderChk_1_Cal [function]
  state SecRwRtStLtwdRtwdHolderChk_1_Cal [function]
  state SecRwRtStLgrstInwdOtwdIsPosChk_1_Cal [function]
  state SecRwRtStLgrstUpwdDnwdIsPosChk_1_Cal [function]
  state SecRwRtStLtwdRtwdIsPosChk_1_Cal [function]
  state SecRwRtStLgrstInwdOtwdTrgtPosSelc_1_Cal [function]
  state SecRwRtStLgrstUpwdDnwdTrgtPosSelc_1_Cal [function]
  state SecRwRtStLtwdRtwdTrgtPosSelc_1_Cal [function]
  state SecRwRtStZeroCtrl_1_Cal [function]
  state SecRwRtStZeroHolderChk_1_Cal [function]
  state SecRwRtStZeroIsPosChk_1_Cal [function]
  state SecRwRtStZeroTrgtPosSelc_1_Cal [function]
  (default) -> (junction 42)
  (junction 42) -> (junction 44) : {
      | SecRwRtStChldLckChk_Cal();
      | SecRwRtStHeightChk_Cal();
      | SecRwRtStOccupyChk_Cal();
      | SecRwRtStArmScrnTrgtPosSelc_1_Cal();
      | SecRwRtStArmScrnIsPosChk_1_Cal();
      | SecRwRtStArmScrnHolderChk_1_Cal();
      | SecRwRtStArmScrnCtrl_1_Cal();
      | SecRwRtStBkReclnTrgtPosSelc_1_Cal();
      | SecRwRtStBkReclnIsPosChk_1_Cal();
      | SecRwRtStBkReclnHolderChk_1_Cal();
      | SecRwRtStBkReclnCtrl_1_Cal();
      | SecRwRtStFtrstTrgtPosSelc_1_Cal();
      | SecRwRtStFtrstIsPosChk_1_Cal();
      | SecRwRtStFtrstHolderChk_1_Cal();
      | SecRwRtStFtrstCtrl_1_Cal();
      | SecRwRtStFwdBkwdTrgtPosSelc_1_Cal();
      | SecRwRtStFwdBkwdIsPosChk_1_Cal();
      | SecRwRtStFwdBkwdHolderChk_1_Cal();
      | SecRwRtStFwdBkwdCtrl_1_Cal();
      | SecRwRtStFwdBkwdSpdCtrl_1_Cal();
      | SecRwRtStHdrstFwdBkwdTrgtPosSelc_1_Cal();
      | SecRwRtStHdrstFwdBkwdIsPosChk_1_Cal();
      | SecRwRtStHdrstFwdBkwdHolderChk_1_Cal();
      | SecRwRtStHdrstFwdBkwdCtrl_1_Cal();
      | SecRwRtStHdrstUpwdDnwdTrgtPosSelc_1_Cal();
      | SecRwRtStHdrstUpwdDnwdIsPosChk_1_Cal();
      | SecRwRtStHdrstUpwdDnwdHolderChk_1_Cal();
      | SecRwRtStHdrstUpwdDnwdCtrl_1_Cal();
      | SecRwRtStLgrstInwdOtwdTrgtPosSelc_1_Cal();
      | SecRwRtStLgrstInwdOtwdIsPosChk_1_Cal();
      | SecRwRtStLgrstInwdOtwdHolderChk_1_Cal();
      | SecRwRtStLgrstInwdOtwdCtrl_1_Cal();
      | SecRwRtStLgrstUpwdDnwdTrgtPosSelc_1_Cal();
      | SecRwRtStLgrstUpwdDnwdIsPosChk_1_Cal();
      | SecRwRtStLgrstUpwdDnwdHolderChk_1_Cal();
      | SecRwRtStLgrstUpwdDnwdCtrl_1_Cal();
      | SecRwRtStLtwdRtwdTrgtPosSelc_1_Cal();
      | SecRwRtStLtwdRtwdIsPosChk_1_Cal();
      | SecRwRtStLtwdRtwdHolderChk_1_Cal();
      | SecRwRtStLtwdRtwdCtrl_1_Cal();
      | SecRwRtStZeroTrgtPosSelc_1_Cal();
      | SecRwRtStZeroIsPosChk_1_Cal();
      | SecRwRtStZeroHolderChk_1_Cal();
      | SecRwRtStZeroCtrl_1_Cal();
      | SecRwRtStRclCmdSrvCal_1_Cal();
      | }
